simulink library "AVE_Library"  (R2025b)
settings: Solver=VariableStepAuto  StartTime=0.0  StopTime=10.0  RelTol=1e-3
undefined symbols (not defined in the file or in its folder): DiscIntNeverNeededParam
libraries: simulink x44, etargetslib x18, $bdroot x13, GenericTarget x2
(part 3 of 5)

== system AVE_Library/Essential/Signal Logics/Index Of Latest Trigger ==
  vecTrigger : Inport
  Detect Rise Positive : simulink/Logic and Bit Operations/Detect Rise Positive  vinit=0  OutDataTypeStr=boolean
  MATLAB Function : MATLAB Function  TreatAsAtomicUnit=on
  idx : Outport
  wires:
  MATLAB Function/1(value) -> idx/1
  Detect Rise Positive/1 -> MATLAB Function/1(buttons)
  vecTrigger/1 -> Detect Rise Positive/1

== system AVE_Library/Essential/Signal Logics/Index To Enable Vector ==
  idx : Inport  OutDataTypeStr=uint8
  AND : Logic  AllPortsSameDT=off  OutDataTypeStr=boolean
  Cast To Boolean : DataTypeConversion  OutDataTypeStr=boolean  SaturateOnIntegerOverflow=off  RndMeth=Floor
  Compare To Constant : simulink/Logic and Bit Operations/Compare To Constant  relop=<  const=uint8(outputSize)  OutDataTypeStr=boolean
  Compare To Zero : simulink/Logic and Bit Operations/Compare To Zero  relop=>=  OutDataTypeStr=boolean
  Constant43 : Constant  Value=zeros(outputSize,1)  OutDataTypeStr=uint8
  Enabled Subsystem : Subsystem  TreatAsAtomicUnit=on
  Switch : Switch  Criteria=u2 ~= 0  SaturateOnIntegerOverflow=off  InputSameDT=off
  vecEnabled : Outport  OutDataTypeStr=boolean
  wires:
  Cast To Boolean/1 -> vecEnabled/1
  idx/1 -> Compare To Zero/1, Compare To Constant/1, Enabled Subsystem/1(index)
  AND/1 -> Switch/2, Enabled Subsystem/Enable
  Enabled Subsystem/1(vecValue) -> Switch/1
  Compare To Zero/1 -> AND/1
  Switch/1 -> Cast To Boolean/1
  Constant43/1 -> Switch/3
  Compare To Constant/1 -> AND/2

== system AVE_Library/Essential/Signal Logics/Push Buttons To Toggle Switches ==
  pushButtons : Inport  OutDataTypeStr=boolean
  reset : Inport  Port=2  OutDataTypeStr=boolean  PortDimensions=1
  Detect Increase : simulink/Logic and Bit Operations/Detect Increase  vinit=0.0  OutDataTypeStr=boolean
  MATLAB Function : MATLAB Function  TreatAsAtomicUnit=on
  toggleSwitches : Outport  OutDataTypeStr=boolean
  wires:
  Detect Increase/1 -> MATLAB Function/1(riseEvent)
  pushButtons/1 -> Detect Increase/1
  reset/1 -> MATLAB Function/2(resetEvent)
  MATLAB Function/1(output) -> toggleSwitches/1

== system AVE_Library/Essential/Signal Logics/Resetable Index Of Latest Trigger ==
  vecTrigger : Inport
  reset : Inport  Port=2  OutDataTypeStr=boolean  PortDimensions=1
  resetValue : Inport  Port=3  OutDataTypeStr=uint8  PortDimensions=1
  Detect Rise Positive : simulink/Logic and Bit Operations/Detect Rise Positive  vinit=0  OutDataTypeStr=boolean
  MATLAB Function : MATLAB Function  TreatAsAtomicUnit=on
  idx : Outport  OutDataTypeStr=uint8  PortDimensions=1
  wires:
  Detect Rise Positive/1 -> MATLAB Function/1(buttons)
  MATLAB Function/1(value) -> idx/1
  reset/1 -> MATLAB Function/2(reset)
  vecTrigger/1 -> Detect Rise Positive/1
  resetValue/1 -> MATLAB Function/3(resetValue)

== system AVE_Library/Essential/Signal Logics/Resetable Toggle Value Up ==
  triggerUp : Inport  PortDimensions=1
  reset : Inport  Port=2  OutDataTypeStr=boolean  PortDimensions=1
  Detect Rise Positive : simulink/Logic and Bit Operations/Detect Rise Positive  vinit=0  OutDataTypeStr=boolean
  MATLAB Function : MATLAB Function  TreatAsAtomicUnit=on
  value : Outport  OutDataTypeStr=uint8  PortDimensions=1
  wires:
  Detect Rise Positive/1 -> MATLAB Function/1(triggerRise)
  reset/1 -> MATLAB Function/2(reset)
  triggerUp/1 -> Detect Rise Positive/1
  MATLAB Function/1(value) -> value/1

== system AVE_Library/Essential/Signal Logics/Time To Latest Event ==
  event : Inport  OutDataTypeStr=boolean  PortDimensions=1
  steadyClock : Inport  Port=2  OutDataTypeStr=double  Unit=s  PortDimensions=1
  CalculateTimeToLatestEvent : MATLAB Function  TreatAsAtomicUnit=on
  timeToLatestEvent : Outport  OutDataTypeStr=double  Unit=s  PortDimensions=1
  wires:
  event/1 -> CalculateTimeToLatestEvent/1(event)
  steadyClock/1 -> CalculateTimeToLatestEvent/2(t)
  CalculateTimeToLatestEvent/1(timeToLatestEvent) -> timeToLatestEvent/1

== system AVE_Library/Essential/Signal Logics/Toggle Value Up ==
  triggerUp : Inport  PortDimensions=1
  Detect Rise Positive : simulink/Logic and Bit Operations/Detect Rise Positive  vinit=0  OutDataTypeStr=boolean
  Toggle : Subsystem  TreatAsAtomicUnit=on
  value : Outport
  wires:
  Detect Rise Positive/1 -> Toggle/Enable
  triggerUp/1 -> Detect Rise Positive/1
  Toggle/1(value) -> value/1

== system AVE_Library/Essential/Signal Logics/Toggle Value Up Down ==
  triggerUp : Inport  PortDimensions=1
  triggerDown : Inport  Port=2  PortDimensions=1
  Detect Rise Positive1 : simulink/Logic and Bit Operations/Detect Rise Positive  vinit=0  OutDataTypeStr=boolean
  Detect Rise Positive2 : simulink/Logic and Bit Operations/Detect Rise Positive  vinit=0  OutDataTypeStr=boolean
  MATLAB Function : MATLAB Function  TreatAsAtomicUnit=on
  value : Outport  OutDataTypeStr=uint8  PortDimensions=1
  wires:
  triggerUp/1 -> Detect Rise Positive1/1
  Detect Rise Positive2/1 -> MATLAB Function/2(down)
  MATLAB Function/1(y) -> value/1
  triggerDown/1 -> Detect Rise Positive2/1
  Detect Rise Positive1/1 -> MATLAB Function/1(up)

== system AVE_Library/Essential/Signal Logics/Trigger Generator ==
  note: required for safe comparison of doubles
  triggerPeriod : Inport  OutDataTypeStr=double  Unit=s  PortDimensions=1
  reset : Inport  Port=2  OutDataTypeStr=boolean  PortDimensions=1
  Add : Sum  Inputs=-+
  Bias : Bias  Bias=-1.0e-12  SaturateOnIntegerOverflow=off
  Digital Clock : DigitalClock  SampleTime=SampleTime
  Enabled Subsystem : Subsystem  TreatAsAtomicUnit=on
  OR : Logic  Operator=OR  AllPortsSameDT=off  OutDataTypeStr=boolean
  Relational Operator : RelationalOperator  OutDataTypeStr=boolean  RndMeth=Simplest  InputSameDT=off
  Unit Delay : UnitDelay  SampleTime=SampleTime  HasFrameUpgradeWarning=on
  trigger : Outport  OutDataTypeStr=boolean  PortDimensions=1
  wires:
  Unit Delay/1 -> Add/1
  OR/1 -> Enabled Subsystem/Enable, trigger/1
  Enabled Subsystem/1(offsetTime) -> Unit Delay/1  "t0"
  Digital Clock/1 -> Add/2, Enabled Subsystem/1(time)
  Add/1 -> Relational Operator/1
  triggerPeriod/1 -> Bias/1
  Relational Operator/1 -> OR/2
  reset/1 -> OR/1
  Bias/1 -> Relational Operator/2

== system AVE_Library/Essential/Transformation/Euler ZYX To Quaternion ==
  roll : Inport  OutDataTypeStr=double  Unit=rad  PortDimensions=1
  pitch : Inport  Port=2  OutDataTypeStr=double  Unit=rad  PortDimensions=1
  yaw : Inport  Port=3  OutDataTypeStr=double  Unit=rad  PortDimensions=1
  MATLAB Function1 : MATLAB Function  TreatAsAtomicUnit=on
  q_b2n : Outport  OutDataTypeStr=double  PortDimensions=4
  wires:
  yaw/1 -> MATLAB Function1/3(yaw)
  MATLAB Function1/1(q) -> q_b2n/1
  roll/1 -> MATLAB Function1/1(roll)
  pitch/1 -> MATLAB Function1/2(pitch)

== system AVE_Library/Essential/Transformation/Euler ZYX To Rotation Matrix ==
  roll : Inport  OutDataTypeStr=double  Unit=rad  PortDimensions=1
  pitch : Inport  Port=2  OutDataTypeStr=double  Unit=rad  PortDimensions=1
  yaw : Inport  Port=3  OutDataTypeStr=double  Unit=rad  PortDimensions=1
  MATLAB Function : MATLAB Function  TreatAsAtomicUnit=on
  Rb2n : Outport  OutDataTypeStr=double  PortDimensions=[3 3]
  wires:
  yaw/1 -> MATLAB Function/3(yaw)
  MATLAB Function/1(R) -> Rb2n/1
  pitch/1 -> MATLAB Function/2(pitch)
  roll/1 -> MATLAB Function/1(roll)

== system AVE_Library/Essential/Transformation/LLA To NED ==
  lat : Inport  OutDataTypeStr=double  Unit=rad
  lon : Inport  Port=2  OutDataTypeStr=double  Unit=rad
  alt : Inport  Port=3  OutDataTypeStr=double  Unit=m
  originLat : Inport  Port=4  OutDataTypeStr=double  Unit=rad  PortDimensions=1
  originLon : Inport  Port=5  OutDataTypeStr=double  Unit=rad  PortDimensions=1
  originAlt : Inport  Port=6  OutDataTypeStr=double  Unit=m  PortDimensions=1
  MATLAB Function : MATLAB Function  TreatAsAtomicUnit=on
  N : Outport  OutDataTypeStr=double  Unit=m  VectorParamsAs1DForOutWhenUnconnected=off
  E : Outport  Port=2  OutDataTypeStr=double  Unit=m  VectorParamsAs1DForOutWhenUnconnected=off
  D : Outport  Port=3  OutDataTypeStr=double  Unit=m  VectorParamsAs1DForOutWhenUnconnected=off
  wires:
  lon/1 -> MATLAB Function/2(lon)
  originLat/1 -> MATLAB Function/4(originLat)
  MATLAB Function/2(E) -> E/1
  originLon/1 -> MATLAB Function/5(originLon)
  lat/1 -> MATLAB Function/1(lat)
  MATLAB Function/1(N) -> N/1
  alt/1 -> MATLAB Function/3(alt)
  originAlt/1 -> MATLAB Function/6(originAlt)
  MATLAB Function/3(D) -> D/1

== system AVE_Library/Essential/Transformation/LLA To NED Vector ==
  positionLLA : Inport  OutDataTypeStr=double
  originLLA : Inport  Port=2  OutDataTypeStr=double
  MATLAB Function : MATLAB Function  TreatAsAtomicUnit=on
  positionNED : Outport  OutDataTypeStr=double  Unit=m
  wires:
  positionLLA/1 -> MATLAB Function/1(positionLLA)
  MATLAB Function/1(NED) -> positionNED/1
  originLLA/1 -> MATLAB Function/2(originLLA)

== system AVE_Library/Essential/Transformation/NED To LLA ==
  N : Inport  OutDataTypeStr=double  Unit=m
  E : Inport  Port=2  OutDataTypeStr=double  Unit=m
  D : Inport  Port=3  OutDataTypeStr=double  Unit=m
  originLat : Inport  Port=4  OutDataTypeStr=double  Unit=rad  PortDimensions=1
  originLon : Inport  Port=5  OutDataTypeStr=double  Unit=rad  PortDimensions=1
  originAlt : Inport  Port=6  OutDataTypeStr=double  Unit=m  PortDimensions=1
  MATLAB Function : MATLAB Function  TreatAsAtomicUnit=on
  lat : Outport  OutDataTypeStr=double  Unit=rad
  lon : Outport  Port=2  OutDataTypeStr=double  Unit=rad
  alt : Outport  Port=3  OutDataTypeStr=double  Unit=m
  wires:
  MATLAB Function/3(alt) -> alt/1
  MATLAB Function/2(lon) -> lon/1
  MATLAB Function/1(lat) -> lat/1
  N/1 -> MATLAB Function/1(N)
  E/1 -> MATLAB Function/2(E)
  D/1 -> MATLAB Function/3(D)
  originLat/1 -> MATLAB Function/4(originLat)
  originLon/1 -> MATLAB Function/5(originLon)
  originAlt/1 -> MATLAB Function/6(originAlt)

== system AVE_Library/Essential/Transformation/NED To LLA Vector ==
  positionNED : Inport  OutDataTypeStr=double  Unit=m
  originLLA : Inport  Port=2  OutDataTypeStr=double
  MATLAB Function : MATLAB Function  TreatAsAtomicUnit=on
  positionLLA : Outport
  wires:
  positionNED/1 -> MATLAB Function/1(positionNED)
  originLLA/1 -> MATLAB Function/2(originLLA)
  MATLAB Function/1(positionLLA) -> positionLLA/1

== system AVE_Library/Essential/Transformation/Quaternion To Euler ZYX ==
  q_b2n : Inport  OutDataTypeStr=double  PortDimensions=4
  MATLAB Function : MATLAB Function  TreatAsAtomicUnit=on
  roll : Outport  OutDataTypeStr=double  Unit=rad  PortDimensions=1
  pitch : Outport  Port=2  OutDataTypeStr=double  Unit=rad  PortDimensions=1
  yaw : Outport  Port=3  OutDataTypeStr=double  Unit=rad  PortDimensions=1
  wires:
  MATLAB Function/1(roll) -> roll/1
  q_b2n/1 -> MATLAB Function/1(q)
  MATLAB Function/3(yaw) -> yaw/1
  MATLAB Function/2(pitch) -> pitch/1

== system AVE_Library/Essential/Transformation/Quaternion To Rotation Matrix ==
  q_b2n : Inport  OutDataTypeStr=double  PortDimensions=4
  MATLAB Function : MATLAB Function  TreatAsAtomicUnit=on
  Cb2n : Outport  OutDataTypeStr=double
  wires:
  q_b2n/1 -> MATLAB Function/1(qb2n)
  MATLAB Function/1(matCb2n) -> Cb2n/1

== system AVE_Library/Essential/Transformation/Transform Sensor Euler ZYX ==
  rollSensor : Inport  OutDataTypeStr=double  Unit=rad  PortDimensions=1
  pitchSensor : Inport  Port=2  OutDataTypeStr=double  Unit=rad  PortDimensions=1
  yawSensor : Inport  Port=3  OutDataTypeStr=double  Unit=rad  PortDimensions=1
  R_b2s : Inport  Port=4  OutDataTypeStr=double  PortDimensions=[3 3]
  MATLAB Function : MATLAB Function  TreatAsAtomicUnit=on
  rollBody : Outport  OutDataTypeStr=double  Unit=rad  PortDimensions=1
  pitchBody : Outport  Port=2  OutDataTypeStr=double  Unit=rad  PortDimensions=1
  yawBody : Outport  Port=3  OutDataTypeStr=double  Unit=rad  PortDimensions=1
  wires:
  rollSensor/1 -> MATLAB Function/1(rollSensor)
  MATLAB Function/2(pitchBody) -> pitchBody/1
  R_b2s/1 -> MATLAB Function/4(R_b2s)
  MATLAB Function/1(rollBody) -> rollBody/1
  pitchSensor/1 -> MATLAB Function/2(pitchSensor)
  yawSensor/1 -> MATLAB Function/3(yawSensor)
  MATLAB Function/3(yawBody) -> yawBody/1

== system AVE_Library/Essential/Transformation/Transform Sensor Position LLA ==
  latSensor : Inport  OutDataTypeStr=double  Unit=rad  PortDimensions=1
  lonSensor : Inport  Port=2  OutDataTypeStr=double  Unit=rad  PortDimensions=1
  altSensor : Inport  Port=3  OutDataTypeStr=double  Unit=m  PortDimensions=1
  R_b2n : Inport  Port=4  OutDataTypeStr=double  PortDimensions=[3 3]
  r_b2s : Inport  Port=5  OutDataTypeStr=double  PortDimensions=3
  MATLAB Function : MATLAB Function  TreatAsAtomicUnit=on
  latBody : Outport  OutDataTypeStr=double  Unit=rad  PortDimensions=1
  lonBody : Outport  Port=2  OutDataTypeStr=double  Unit=rad  PortDimensions=1
  altBody : Outport  Port=3  OutDataTypeStr=double  Unit=m  PortDimensions=1
  wires:
  altSensor/1 -> MATLAB Function/3(altSensor)
  MATLAB Function/3(altBody) -> altBody/1
  MATLAB Function/2(lonBody) -> lonBody/1
  MATLAB Function/1(latBody) -> latBody/1
  latSensor/1 -> MATLAB Function/1(latSensor)
  lonSensor/1 -> MATLAB Function/2(lonSensor)
  R_b2n/1 -> MATLAB Function/4(R_b2n)
  r_b2s/1 -> MATLAB Function/5(r_b2s)

== system AVE_Library/Essential/Transformation/Transform Sensor Quaternion WXYZ ==
  quaternionSensor : Inport  OutDataTypeStr=double  PortDimensions=4
  R_b2s : Inport  Port=2  OutDataTypeStr=double  PortDimensions=[3 3]
  MATLAB Function : MATLAB Function  TreatAsAtomicUnit=on
  quaternionBody : Outport  OutDataTypeStr=double  PortDimensions=4
  wires:
  MATLAB Function/1(quaternionBody) -> quaternionBody/1
  quaternionSensor/1 -> MATLAB Function/1(quaternionSensor)
  R_b2s/1 -> MATLAB Function/2(R_b2s)

== system AVE_Library/Essential/Transformation/Transform Sensor Velocity PQR ==
  pSensor : Inport  OutDataTypeStr=double  Unit=rad/s  PortDimensions=1
  qSensor : Inport  Port=2  OutDataTypeStr=double  Unit=rad/s  PortDimensions=1
  rSensor : Inport  Port=3  OutDataTypeStr=double  Unit=rad/s  PortDimensions=1
  R_b2s : Inport  Port=4  OutDataTypeStr=double  PortDimensions=[3 3]
  MATLAB Function : MATLAB Function  TreatAsAtomicUnit=on
  pBody : Outport  OutDataTypeStr=double  Unit=rad/s  PortDimensions=1
  qBody : Outport  Port=2  OutDataTypeStr=double  Unit=rad/s  PortDimensions=1
  rBody : Outport  Port=3  OutDataTypeStr=double  Unit=rad/s  PortDimensions=1
  wires:
  MATLAB Function/3(rBody) -> rBody/1
  rSensor/1 -> MATLAB Function/3(rSensor)
  qSensor/1 -> MATLAB Function/2(qSensor)
  MATLAB Function/1(pBody) -> pBody/1
  R_b2s/1 -> MATLAB Function/4(R_b2s)
  MATLAB Function/2(qBody) -> qBody/1
  pSensor/1 -> MATLAB Function/1(pSensor)

== system AVE_Library/Essential/Transformation/Transform Sensor Velocity UVW ==
  uSensor : Inport  OutDataTypeStr=double  Unit=m/s  PortDimensions=1
  vSensor : Inport  Port=2  OutDataTypeStr=double  Unit=m/s  PortDimensions=1
  wSensor : Inport  Port=3  OutDataTypeStr=double  Unit=m/s  PortDimensions=1
  R_b2s : Inport  Port=4  OutDataTypeStr=double  PortDimensions=[3 3]
  r_b2s : Inport  Port=5  OutDataTypeStr=double  Unit=m  PortDimensions=3
  pqr : Inport  Port=6  OutDataTypeStr=double  Unit=rad/s  PortDimensions=3
  MATLAB Function : MATLAB Function  TreatAsAtomicUnit=on
  uBody : Outport  OutDataTypeStr=double  Unit=m/s  PortDimensions=1
  vBody : Outport  Port=2  OutDataTypeStr=double  Unit=m/s  PortDimensions=1
  wBody : Outport  Port=3  OutDataTypeStr=double  Unit=m/s  PortDimensions=1
  wires:
  uSensor/1 -> MATLAB Function/1(uSensor)
  MATLAB Function/2(vBody) -> vBody/1
  R_b2s/1 -> MATLAB Function/4(R_b2s)
  MATLAB Function/1(uBody) -> uBody/1
  pqr/1 -> MATLAB Function/6(pqr)
  vSensor/1 -> MATLAB Function/2(vSensor)
  r_b2s/1 -> MATLAB Function/5(r_b2s)
  wSensor/1 -> MATLAB Function/3(wSensor)
  MATLAB Function/3(wBody) -> wBody/1

== system AVE_Library/Essential/Transformation/Yaw To Rotation Matrix ==
  yaw : Inport  OutDataTypeStr=double  Unit=rad  PortDimensions=1
  MATLAB Function : MATLAB Function  TreatAsAtomicUnit=on
  Rb2n : Outport  OutDataTypeStr=double  PortDimensions=[2 2]
  wires:
  MATLAB Function/1(R) -> Rb2n/1
  yaw/1 -> MATLAB Function/1(yaw)

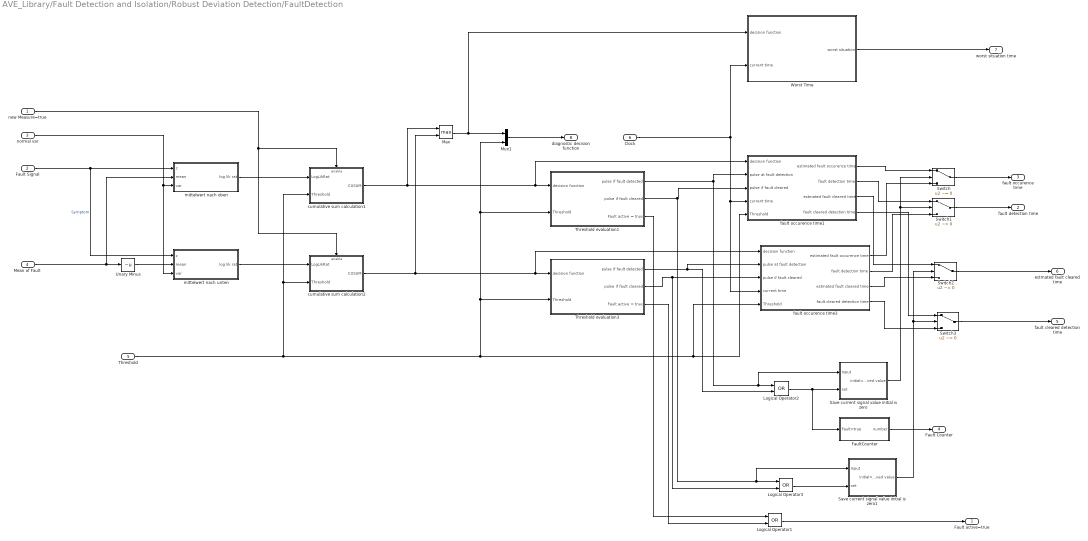
== system AVE_Library/Fault Detection and Isolation/Robust Deviation Detection/FaultDetection ==
  new Measure=true : Inport
  Fault Signal : Inport  Port=2
  normal var : Inport  Port=3
  Mean of Fault : Inport  Port=4
  Threshold : Inport  Port=5
  Clock : Inport  Port=6
  FaultCounter : Subsystem
  Logical Operator1 : Logic  Operator=OR  AllPortsSameDT=off  OutDataTypeStr=boolean
  Logical Operator2 : Logic  Operator=OR  AllPortsSameDT=off  OutDataTypeStr=boolean
  Logical Operator3 : Logic  Operator=OR  AllPortsSameDT=off  OutDataTypeStr=boolean
  Max : MinMax  Function=max  Inputs=2
  Mux1 : Mux  Inputs=2
  Save current signal value initial is zero : Subsystem  mask(save current signal value){}
      mask help:
      | If set is not zero, the input is feed throug to the output.
      | If set is zero, the output remains the last intput value when set was not zero.
      | Initial value is zero.
  Save current signal value initial is zero1 : Subsystem  mask(save current signal value){}
      mask help:
      | If set is not zero, the input is feed throug to the output.
      | If set is zero, the output remains the last intput value when set was not zero.
      | Initial value is zero.
  Switch{,1..3} (4 alike) : Switch  Criteria=u2 ~= 0  SaturateOnIntegerOverflow=off  InputSameDT=off
  Threshold evaluation1 : Subsystem
  Threshold evaluation3 : Subsystem
  Unary Minus : UnaryMinus
  Worst Time : Subsystem
  cumulative sum calculation1 : Subsystem
  cumulative sum calculation2 : Subsystem
  fault occurence time1 : Subsystem
  fault occurence time3 : Subsystem
  mittelwert nach oben : Subsystem
  mittelwert nach unten : Subsystem
  Fault active=true : Outport  VectorParamsAs1DForOutWhenUnconnected=off
  fault detection time : Outport  Port=2  VectorParamsAs1DForOutWhenUnconnected=off
  fault occurence time : Outport  Port=3  VectorParamsAs1DForOutWhenUnconnected=off
  Fault Counter : Outport  Port=4  VectorParamsAs1DForOutWhenUnconnected=off
  fault cleared detection time : Outport  Port=5  VectorParamsAs1DForOutWhenUnconnected=off
  estmated fault cleared time : Outport  Port=6  VectorParamsAs1DForOutWhenUnconnected=off
  worst situation time : Outport  Port=7  VectorParamsAs1DForOutWhenUnconnected=off
  diagnostic decision function : Outport  Port=8  VectorParamsAs1DForOutWhenUnconnected=off
  wires:
  mittelwert nach unten/1(log lik rat) -> cumulative sum calculation2/1(LogLikRat)
  mittelwert nach oben/1(log lik rat) -> cumulative sum calculation1/1(LogLikRat)
  Worst Time/1(worst situation) -> worst situation time/1
  Switch3/1 -> fault cleared detection time/1
  Switch2/1 -> estmated fault cleared time/1
  fault occurence time3/3(estmated fault cleared time) -> Switch2/3
  fault occurence time3/4(fault cleared detection time) -> Switch3/3
  fault occurence time1/4(fault cleared detection time) -> Switch3/1
  fault occurence time1/3(estmated fault cleared time) -> Switch2/1
  Save current signal value initial is zero1/1(initial=0  saved value) -> Switch3/2, Switch2/2
  Threshold evaluation1/2(pulse if fault cleared) -> fault occurence time1/3(pulse if fault cleared), Logical Operator3/1, Save current signal value initial is zero1/1(Input)
  Logical Operator3/1 -> Save current signal value initial is zero1/2(set)
  Threshold evaluation3/2(pulse if fault cleared) -> Logical Operator3/2, fault occurence time3/3(pulse if fault cleared)
  FaultCounter/1(number) -> Fault Counter/1
  Mux1/1 -> diagnostic decision function/1
  Threshold/1 -> cumulative sum calculation2/2(Threshold), cumulative sum calculation1/2(Threshold), Mux1/2, Threshold evaluation1/2(Threshold), Threshold evaluation3/2(Threshold), fault occurence time1/5(Threshold), fault occurence time3/5(Threshold)
  Max/1 -> Mux1/1, Worst Time/1(decision function)
  Logical Operator1/1 -> Fault active=true/1
  fault occurence time3/2(fault detection time) -> Switch1/3
  fault occurence time1/2(fault detection time) -> Switch1/1
  fault occurence time3/1(estimated fault occurence time) -> Switch/3
  fault occurence time1/1(estimated fault occurence time) -> Switch/1
  Threshold evaluation3/3(Fault active = true) -> Logical Operator1/2
  Threshold evaluation1/3(Fault active = true) -> Logical Operator1/1
  Threshold evaluation3/1(pulse if fault detected) -> Logical Operator2/2, fault occurence time3/2(pulse at fault detection)
  new Measure=true/1 -> cumulative sum calculation1/Enable, cumulative sum calculation2/Enable
  cumulative sum calculation2/1(CUSUM) -> Max/2, fault occurence time3/1(decision function), Threshold evaluation3/1(decision function)
  Save current signal value initial is zero/1(initial=0  saved value) -> Switch1/2, Switch/2
  Logical Operator2/1 -> Save current signal value initial is zero/2(set), FaultCounter/1(Fault=true)
  Threshold evaluation1/1(pulse if fault detected) -> fault occurence time1/2(pulse at fault detection), Save current signal value initial is zero/1(Input), Logical Operator2/1
  Switch1/1 -> fault detection time/1
  Switch/1 -> fault occurence time/1
  cumulative sum calculation1/1(CUSUM) -> Max/1, fault occurence time1/1(decision function), Threshold evaluation1/1(decision function)
  Unary Minus/1 -> mittelwert nach unten/2(mean)
  Clock/1 -> fault occurence time1/4(current time), fault occurence time3/4(current time), Worst Time/2(current time)
  Mean of Fault/1 -> Unary Minus/1, mittelwert nach oben/2(mean)
  Fault Signal/1 -> mittelwert nach unten/1(z), mittelwert nach oben/1(z)  "Symptom"
  normal var/1 -> mittelwert nach oben/3(var), mittelwert nach unten/3(var)

== system AVE_Library/Fault Detection and Isolation/Robust Deviation Detection/mittelwert nach oben ==
  mean : Inport
  z : Inport  Port=2
  var : Inport  Port=3
  Gain2 : Gain  Gain=0.5
  Product1 : Product  Inputs=**/  RndMeth=Zero
  Sum : Sum  Inputs=+-|
  null Vermeiden : Subsystem  mask{kleinsterWert=1e-8}
      mask prompts: kleinsterWert "Null-Mindestabstand"
      mask help:
      | Der Ausgang hält einen vorgegebenen Abstand zu Null.
      | Wenn der Eingang einen Nulldurchlauf hat, springt der Ausgang von +Mindestabstand nach -Mindestabstand, bzw. von -Mindestabstand nach +Mindestabstand. Bei Eingang ==0: Ausgang=+Mindestabstand
  log lik rat : Outport  VectorParamsAs1DForOutWhenUnconnected=off
  wires:
  null Vermeiden/1(non zero) -> Product1/3
  Gain2/1 -> Sum/2
  Sum/1 -> Product1/1
  z/1 -> Sum/1
  Product1/1 -> log lik rat/1
  var/1 -> null Vermeiden/1(value)
  mean/1 -> Gain2/1, Product1/2

== system AVE_Library/Fault Detection and Isolation/Robust Deviation Detection/statistics ==
  measurement value : Inport
  measurement state 1/0 : Inport  Port=2
  n max : Inport  Port=3
  Constant1 : Constant  Value=0
  Messwertzähler : Subsystem
  Subsystem : Subsystem
  var : Outport
  wires:
  measurement state 1/0/1 -> Messwertzähler/1(measurement state), Subsystem/Enable
  Constant1/1 -> Subsystem/1(mean)
  n max/1 -> Messwertzähler/2(n max)
  Messwertzähler/1(number) -> Subsystem/2(n measurements)
  measurement value/1 -> Subsystem/3(measurement)
  Subsystem/1(var) -> var/1

== system AVE_Library/Navigation/Sensor Preprocessing/Butterworth Filter ==
  u : Inport
  T : Inport  Port=2
  Butterworth Low Pass and Derivation : Subsystem  mask(Butterworth Lowpass Filter){n_Ordnung_Butter_Simulink=numPoles, n_Ableitung=numZeros}
      mask prompts: n_Ordnung_Butter_Simulink "Ordnung Tiefpass"; n_Ableitung "Anzahl Ableitungen"
      mask help:
      | Butterworth Lowpass Filter mit variabler Frequenz.
      | Ordnung ist nicht online tunable, dies würde zu variabler Dimension der Matrizen führen.
      mask init:
      | if n_Ableitung==0
      |     nozerosFlag=1;
      |     Nullstellen=0;
      | else
      |     nozerosFlag=0;
      |     Nullstellen=zeros(1,n_Ableitung);
      | end
      | 
      | 
      | if n_Ableitung>n_Ordnung_Butter_Simulink
      |     error('Ordnung muss mindestens so hoch wie Anzahl Ableitungen sein. ')
      | end
      mask Display:
      | %text(.5,.5,'{\itEquation:}  \Sigma \alpha^2 + \beta^2 \rightarrow \infty, \Pi, \phi_3 = {\bfcool}', 'hor','left','texmode','on')
      | %text(0.5, 0.5, ['Butterworth\nLowpass\n n_Ordnung=' num2str(n_Ordnung_Butter_Simulink) '\nn_Ableitungen=' num2str(n_Ableitung) ], 'horizontalAlignment', 'center');
      | text(0.5, 0.5, 'Butterworth\nFilter Design', 'horizontalAlignment', 'center');
  Detect Change : simulink/Logic and Bit Operations/Detect Change  vinit=0  OutDataTypeStr=boolean
  Zustandsraummodell x0=x_t_inf(u=u_t_0) : Subsystem
  y : Outport  VectorParamsAs1DForOutWhenUnconnected=off
  wires:
  Detect Change/1 -> Zustandsraummodell x0=x_t_inf(u=u_t_0)/6(reset)
  T/1 -> Detect Change/1, Butterworth Low Pass and Derivation/1(T)
  Butterworth Low Pass and Derivation/2(B) -> Zustandsraummodell x0=x_t_inf(u=u_t_0)/2(B)
  Zustandsraummodell x0=x_t_inf(u=u_t_0)/1(y) -> y/1
  Butterworth Low Pass and Derivation/4(D) -> Zustandsraummodell x0=x_t_inf(u=u_t_0)/4(D)
  Butterworth Low Pass and Derivation/1(A) -> Zustandsraummodell x0=x_t_inf(u=u_t_0)/1(A)
  Butterworth Low Pass and Derivation/3(C) -> Zustandsraummodell x0=x_t_inf(u=u_t_0)/3(C)
  u/1 -> Zustandsraummodell x0=x_t_inf(u=u_t_0)/5(u)

== system AVE_Library/Navigation/Sensor Preprocessing/Detect Outliers 1D ==
  triggerNewData : Inport  OutDataTypeStr=boolean  PortDimensions=1
  data : Inport  Port=2  OutDataTypeStr=double  PortDimensions=1
  threshold : Inport  Port=3  OutDataTypeStr=double  PortDimensions=1
  maxNumOutliers : Inport  Port=4  OutDataTypeStr=uint32  PortDimensions=1
  Abs2 : Abs  SaturateOnIntegerOverflow=off
  Constant : Constant  OutDataTypeStr=uint32
  MATLAB Function : MATLAB Function  TreatAsAtomicUnit=on
  Max : MinMax  Function=max  Inputs=2
  numberOfOutliers : Outport  OutDataTypeStr=uint32  PortDimensions=1
  wires:
  MATLAB Function/1(numberOfOutliers) -> numberOfOutliers/1
  data/1 -> MATLAB Function/2(data)
  triggerNewData/1 -> MATLAB Function/1(triggerNewData)
  threshold/1 -> Abs2/1
  Abs2/1 -> MATLAB Function/3(threshold)
  Constant/1 -> Max/2
  maxNumOutliers/1 -> Max/1
  Max/1 -> MATLAB Function/4(maxNumOutliers)

== system AVE_Library/Navigation/Sensor Preprocessing/Detect Outliers Angle 1D ==
  triggerNewData : Inport  OutDataTypeStr=boolean  PortDimensions=1
  data : Inport  Port=2  OutDataTypeStr=double  PortDimensions=1
  threshold : Inport  Port=3  OutDataTypeStr=double  PortDimensions=1
  maxNumOutliers : Inport  Port=4  OutDataTypeStr=uint32  PortDimensions=1
  Abs2 : Abs  SaturateOnIntegerOverflow=off
  Constant : Constant  OutDataTypeStr=uint32
  MATLAB Function : MATLAB Function  TreatAsAtomicUnit=on
  Max : MinMax  Function=max  Inputs=2
  numberOfOutliers : Outport  OutDataTypeStr=uint32  PortDimensions=1
  wires:
  Max/1 -> MATLAB Function/4(maxNumOutliers)
  maxNumOutliers/1 -> Max/1
  Constant/1 -> Max/2
  Abs2/1 -> MATLAB Function/3(threshold)
  threshold/1 -> Abs2/1
  triggerNewData/1 -> MATLAB Function/1(triggerNewData)
  data/1 -> MATLAB Function/2(data)
  MATLAB Function/1(numberOfOutliers) -> numberOfOutliers/1

== system AVE_Library/Navigation/Sensor Preprocessing/Detect Outliers GNSS ==
  triggerNewData : Inport  OutDataTypeStr=boolean  PortDimensions=1
  positionLLA : Inport  Port=2  OutDataTypeStr=double  PortDimensions=3
  thresholdHorizontal : Inport  Port=3  OutDataTypeStr=double  Unit=m  PortDimensions=1
  thresholdVertical : Inport  Port=4  OutDataTypeStr=double  Unit=m  PortDimensions=1
  maxNumOutliers : Inport  Port=5  OutDataTypeStr=uint32  PortDimensions=1
  Abs1 : Abs  SaturateOnIntegerOverflow=off
  Abs2 : Abs  SaturateOnIntegerOverflow=off
  Constant : Constant  OutDataTypeStr=uint32
  MATLAB Function : MATLAB Function  TreatAsAtomicUnit=on
  Max : MinMax  Function=max  Inputs=2
  numberOfOutliers : Outport  OutDataTypeStr=uint32  PortDimensions=1
  wires:
  Max/1 -> MATLAB Function/5(maxNumOutliers)
  maxNumOutliers/1 -> Max/1
  Constant/1 -> Max/2
  Abs2/1 -> MATLAB Function/3(thresholdHorizontal)
  thresholdHorizontal/1 -> Abs2/1
  triggerNewData/1 -> MATLAB Function/1(triggerNewData)
  positionLLA/1 -> MATLAB Function/2(positionLLA)
  MATLAB Function/1(numberOfOutliers) -> numberOfOutliers/1
  Abs1/1 -> MATLAB Function/4(thresholdVertical)
  thresholdVertical/1 -> Abs1/1

== system AVE_Library/Navigation/Sensor Preprocessing/Smoothed Quaternion Time Derivative ==
  time : Inport  OutDataTypeStr=double  Unit=s  PortDimensions=1
  trigger : Inport  Port=2  OutDataTypeStr=boolean  PortDimensions=1
  q_b2n : Inport  Port=3  OutDataTypeStr=double  PortDimensions=4
  timeconstant : Inport  Port=4  OutDataTypeStr=double  Unit=s  PortDimensions=1
  Demux : Demux
  Mux : Mux  Inputs=3
  SmoothedOrientationDeviation : MATLAB Function  TreatAsAtomicUnit=on
  pqr : Outport  OutDataTypeStr=double  Unit=rad/s  PortDimensions=3
  wires:
  time/1 -> SmoothedOrientationDeviation/1(time)
  timeconstant/1 -> SmoothedOrientationDeviation/7(T)
  trigger/1 -> SmoothedOrientationDeviation/2(trigger)
  SmoothedOrientationDeviation/2(q) -> Mux/2
  SmoothedOrientationDeviation/1(p) -> Mux/1
  SmoothedOrientationDeviation/3(r) -> Mux/3
  Mux/1 -> pqr/1
  q_b2n/1 -> Demux/1
  Demux/1 -> SmoothedOrientationDeviation/3(qw)
  Demux/2 -> SmoothedOrientationDeviation/4(qx)
  Demux/3 -> SmoothedOrientationDeviation/5(qy)
  Demux/4 -> SmoothedOrientationDeviation/6(qz)

== system AVE_Library/Navigation/Sensor Preprocessing/Triggered Low Pass ==
  time : Inport  OutDataTypeStr=double  Unit=s  PortDimensions=1
  trigger : Inport  Port=2  OutDataTypeStr=boolean  PortDimensions=1
  input : Inport  Port=3  OutDataTypeStr=double
  timeconstant : Inport  Port=4  OutDataTypeStr=double  Unit=s  PortDimensions=1
  TriggeredLowPass : MATLAB Function  TreatAsAtomicUnit=on
  output : Outport  OutDataTypeStr=double
  wires:
  time/1 -> TriggeredLowPass/1(time)
  input/1 -> TriggeredLowPass/3(u)
  timeconstant/1 -> TriggeredLowPass/4(T)
  trigger/1 -> TriggeredLowPass/2(trigger)
  TriggeredLowPass/1(y) -> output/1

== system AVE_Library/Essential/Equations of Motion/Kinematic 6DoF Geographic/Enabled Subsystem ==
  In1 : Inport
  Enable : EnablePort
  Out1 : Outport  VectorParamsAs1DForOutWhenUnconnected=off
  wires:
  In1/1 -> Out1/1

== system AVE_Library/Essential/Network/Swap Double Host To Network/Swap Each Element ==
  in : Inport  Partition=on  PartitionDimension=1  PartitionWidth=1  PartitionOffset=0
  Byte Pack : etargetslib/Byte Pack  datatypes={'double'}  byteAlign=1
  Byte Unpack : etargetslib/Byte Unpack  dimensions={[1]}  datatypes={'double'}  byteAlign=1
  For Each : ForEach  DisableCoverage=on
  Selector : Selector  InputPortWidth=8  IndexOptions=Index vector (dialog)  Indices=[8 7 6 5 4 3 2 1]  OutputSizes=1
  out : Outport  ConcatenationDimension=1
  wires:
  Selector/1 -> Byte Unpack/1
  Byte Pack/1 -> Selector/1
  Byte Unpack/1 -> out/1
  in/1 -> Byte Pack/1

== system AVE_Library/Essential/Network/Swap Float Host To Network/Swap Each Element ==
  in : Inport  Partition=on  PartitionDimension=1  PartitionWidth=1  PartitionOffset=0
  Byte Pack : etargetslib/Byte Pack  datatypes={'single'}  byteAlign=1
  Byte Unpack : etargetslib/Byte Unpack  dimensions={[1]}  datatypes={'single'}  byteAlign=1
  For Each : ForEach  DisableCoverage=on
  Selector : Selector  InputPortWidth=4  IndexOptions=Index vector (dialog)  Indices=[4 3 2 1]  OutputSizes=1
  out : Outport  ConcatenationDimension=1
  wires:
  Selector/1 -> Byte Unpack/1
  Byte Pack/1 -> Selector/1
  Byte Unpack/1 -> out/1
  in/1 -> Byte Pack/1

== system AVE_Library/Essential/Network/Swap Int16 Host To Network/Swap Each Element ==
  in : Inport  Partition=on  PartitionDimension=1  PartitionWidth=1  PartitionOffset=0
  Byte Pack : etargetslib/Byte Pack  datatypes={'int16'}  byteAlign=1
  Byte Unpack : etargetslib/Byte Unpack  dimensions={[1]}  datatypes={'int16'}  byteAlign=1
  For Each : ForEach  DisableCoverage=on
  Selector : Selector  InputPortWidth=2  IndexOptions=Index vector (dialog)  Indices=[2 1]  OutputSizes=1
  out : Outport  ConcatenationDimension=1
  wires:
  Selector/1 -> Byte Unpack/1
  Byte Pack/1 -> Selector/1
  Byte Unpack/1 -> out/1
  in/1 -> Byte Pack/1

== system AVE_Library/Essential/Network/Swap Int32 Host To Network/Swap Each Element ==
  in : Inport  Partition=on  PartitionDimension=1  PartitionWidth=1  PartitionOffset=0
  Byte Pack : etargetslib/Byte Pack  datatypes={'int32'}  byteAlign=1
  Byte Unpack : etargetslib/Byte Unpack  dimensions={[1]}  datatypes={'int32'}  byteAlign=1
  For Each : ForEach  DisableCoverage=on
  Selector : Selector  InputPortWidth=4  IndexOptions=Index vector (dialog)  Indices=[4 3 2 1]  OutputSizes=1
  out : Outport  ConcatenationDimension=1
  wires:
  Selector/1 -> Byte Unpack/1
  Byte Pack/1 -> Selector/1
  Byte Unpack/1 -> out/1
  in/1 -> Byte Pack/1

== system AVE_Library/Essential/Network/Swap Uint16 Host To Network/Swap Each Element ==
  in : Inport  Partition=on  PartitionDimension=1  PartitionWidth=1  PartitionOffset=0
  Byte Pack : etargetslib/Byte Pack  datatypes={'uint16'}  byteAlign=1
  Byte Unpack : etargetslib/Byte Unpack  dimensions={[1]}  datatypes={'uint16'}  byteAlign=1
  For Each : ForEach  DisableCoverage=on
  Selector : Selector  InputPortWidth=2  IndexOptions=Index vector (dialog)  Indices=[2 1]  OutputSizes=1
  out : Outport  ConcatenationDimension=1
  wires:
  Selector/1 -> Byte Unpack/1
  Byte Pack/1 -> Selector/1
  Byte Unpack/1 -> out/1
  in/1 -> Byte Pack/1

== system AVE_Library/Essential/Network/Swap Uint32 Host To Network/Swap Each Element ==
  in : Inport  Partition=on  PartitionDimension=1  PartitionWidth=1  PartitionOffset=0
  Byte Pack : etargetslib/Byte Pack  datatypes={'uint32'}  byteAlign=1
  Byte Unpack : etargetslib/Byte Unpack  dimensions={[1]}  datatypes={'uint32'}  byteAlign=1
  For Each : ForEach  DisableCoverage=on
  Selector : Selector  InputPortWidth=4  IndexOptions=Index vector (dialog)  Indices=[4 3 2 1]  OutputSizes=1
  out : Outport  ConcatenationDimension=1
  wires:
  in/1 -> Byte Pack/1
  Byte Unpack/1 -> out/1
  Byte Pack/1 -> Selector/1
  Selector/1 -> Byte Unpack/1

== system AVE_Library/Essential/Signal Logics/Index To Enable Vector/Enabled Subsystem ==
  index : Inport
  Enable : EnablePort
  Assignment : Assignment  IndexMode=Zero-based  DiagnosticForDimensions=Warning  IndexOptions=Index vector (port)  Indices=1  OutputSizes=1
  Constant43 : Constant  Value=zeros(outputSize,1)  OutDataTypeStr=uint8
  Constant44 : Constant  OutDataTypeStr=uint8
  vecValue : Outport
  wires:
  Assignment/1 -> vecValue/1
  Constant43/1 -> Assignment/1
  index/1 -> Assignment/3
  Constant44/1 -> Assignment/2

== system AVE_Library/Essential/Signal Logics/Toggle Value Up/Toggle ==
  Enable : EnablePort
  Bias : Bias  Bias=uint8(1)  SaturateOnIntegerOverflow=off
  Compare To Constant : simulink/Logic and Bit Operations/Compare To Constant  relop=<=  const=uint8(maxValue)  OutDataTypeStr=boolean
  Constant : Constant  Value=0  OutDataTypeStr=uint8
  Switch : Switch  Criteria=u2 ~= 0  SaturateOnIntegerOverflow=off  InputSameDT=off
  Unit Delay : UnitDelay  InitialCondition=uint8(0)  SampleTime=-1  HasFrameUpgradeWarning=on
  value : Outport  OutDataTypeStr=uint8  PortDimensions=1
  wires:
  Switch/1 -> Unit Delay/1, value/1
  Constant/1 -> Switch/3
  Compare To Constant/1 -> Switch/2
  Bias/1 -> Switch/1, Compare To Constant/1
  Unit Delay/1 -> Bias/1

== system AVE_Library/Essential/Signal Logics/Trigger Generator/Enabled Subsystem ==
  time : Inport
  Enable : EnablePort
  offsetTime : Outport
  wires:
  time/1 -> offsetTime/1

== system AVE_Library/Fault Detection and Isolation/Robust Deviation Detection/FaultDetection/FaultCounter ==
  Fault=true : Inport
  Data Type Conversion : DataTypeConversion  OutDataTypeStr=uint32  SaturateOnIntegerOverflow=off  RndMeth=Floor
  Memory : Memory  InheritSampleTime=on
  Sum : Sum  Inputs=|++
  number : Outport
  wires:
  Memory/1 -> Sum/1
  Sum/1 -> Memory/1, number/1
  Fault=true/1 -> Data Type Conversion/1
  Data Type Conversion/1 -> Sum/2

== system AVE_Library/Fault Detection and Isolation/Robust Deviation Detection/FaultDetection/Save current signal value initial is zero ==
  Input : Inport
  set : Inport  Port=2
  Init : Switch  Criteria=u2 ~= 0  OutDataTypeStr=Inherit: Inherit via back propagation  ZeroCross=off  SaturateOnIntegerOverflow=off  InputSameDT=off
  Memory : Memory  InheritSampleTime=on
  Reset : Switch  Criteria=u2 ~= 0  OutDataTypeStr=Inherit: Inherit via back propagation  ZeroCross=off  SaturateOnIntegerOverflow=off  InputSameDT=off
  initial=0  saved value : Outport  VectorParamsAs1DForOutWhenUnconnected=off
  wires:
  set/1 -> Reset/2, Init/2
  Memory/1 -> Init/3
  Init/1 -> initial=0  saved value/1, Reset/3
  Reset/1 -> Memory/1
  Input/1 -> Reset/1, Init/1

== system AVE_Library/Fault Detection and Isolation/Robust Deviation Detection/FaultDetection/Save current signal value initial is zero1 ==
  Input : Inport
  set : Inport  Port=2
  Init : Switch  Criteria=u2 ~= 0  OutDataTypeStr=Inherit: Inherit via back propagation  ZeroCross=off  SaturateOnIntegerOverflow=off  InputSameDT=off
  Memory : Memory  InheritSampleTime=on
  Reset : Switch  Criteria=u2 ~= 0  OutDataTypeStr=Inherit: Inherit via back propagation  ZeroCross=off  SaturateOnIntegerOverflow=off  InputSameDT=off
  initial=0  saved value : Outport  VectorParamsAs1DForOutWhenUnconnected=off
  wires:
  Input/1 -> Init/1, Reset/1
  Reset/1 -> Memory/1
  Init/1 -> Reset/3, initial=0  saved value/1
  Memory/1 -> Init/3
  set/1 -> Init/2, Reset/2

== system AVE_Library/Fault Detection and Isolation/Robust Deviation Detection/FaultDetection/Threshold evaluation1 ==
  decision function : Inport
  Threshold : Inport  Port=2
  Compare To Zero : simulink/Logic and Bit Operations/Compare To Zero  relop===  OutDataTypeStr=boolean
  Detect Decrease : simulink/Logic and Bit Operations/Detect Decrease  vinit=0.0  OutDataTypeStr=boolean
  Detect Increase : simulink/Logic and Bit Operations/Detect Increase  vinit=0.0  OutDataTypeStr=boolean
  Detect Increase1 : simulink/Logic and Bit Operations/Detect Increase  vinit=0.0  OutDataTypeStr=boolean
  Detect Increase2 : simulink/Logic and Bit Operations/Detect Increase  vinit=0.0  OutDataTypeStr=boolean
  FehlerSpeicher : Subsystem  mask(save current signal value){}
      mask help:
      | If set is not zero, the input is feed throug to the output.
      | If set is zero, the output remains the last intput value when set was not zero.
      | Initial value is zero.
  OR : Logic  Operator=OR  AllPortsSameDT=off  OutDataTypeStr=boolean
  decisionfunction crosses threshold : RelationalOperator  OutDataTypeStr=boolean  InputSameDT=off
  pulse if fault detected : Outport  VectorParamsAs1DForOutWhenUnconnected=off
  pulse if fault cleared : Outport  Port=2  VectorParamsAs1DForOutWhenUnconnected=off
  Fault active = true : Outport  Port=3  VectorParamsAs1DForOutWhenUnconnected=off
  wires:
  Detect Decrease/1 -> pulse if fault cleared/1
  Detect Increase2/1 -> pulse if fault detected/1
  FehlerSpeicher/1(initial=0  saved value) -> Detect Increase2/1, Detect Decrease/1, Fault active = true/1
  Detect Increase1/1 -> OR/1
  Detect Increase/1 -> OR/2, FehlerSpeicher/1(Input)
  OR/1 -> FehlerSpeicher/2(set)
  Compare To Zero/1 -> Detect Increase1/1
  Threshold/1 -> decisionfunction crosses threshold/2
  decision function/1 -> decisionfunction crosses threshold/1, Compare To Zero/1
  decisionfunction crosses threshold/1 -> Detect Increase/1

== system AVE_Library/Fault Detection and Isolation/Robust Deviation Detection/FaultDetection/Threshold evaluation3 ==
  decision function : Inport
  Threshold : Inport  Port=2
  Compare To Zero : simulink/Logic and Bit Operations/Compare To Zero  relop===  OutDataTypeStr=boolean
  Detect Decrease : simulink/Logic and Bit Operations/Detect Decrease  vinit=0.0  OutDataTypeStr=boolean
  Detect Increase : simulink/Logic and Bit Operations/Detect Increase  vinit=0.0  OutDataTypeStr=boolean
  Detect Increase1 : simulink/Logic and Bit Operations/Detect Increase  vinit=0.0  OutDataTypeStr=boolean
  Detect Increase2 : simulink/Logic and Bit Operations/Detect Increase  vinit=0.0  OutDataTypeStr=boolean
  FehlerSpeicher : Subsystem  mask(save current signal value){}
      mask help:
      | If set is not zero, the input is feed throug to the output.
      | If set is zero, the output remains the last intput value when set was not zero.
      | Initial value is zero.
  OR : Logic  Operator=OR  AllPortsSameDT=off  OutDataTypeStr=boolean
  decisionfunction crosses threshold : RelationalOperator  OutDataTypeStr=boolean  InputSameDT=off
  pulse if fault detected : Outport  VectorParamsAs1DForOutWhenUnconnected=off
  pulse if fault cleared : Outport  Port=2  VectorParamsAs1DForOutWhenUnconnected=off
  Fault active = true : Outport  Port=3  VectorParamsAs1DForOutWhenUnconnected=off
  wires:
  decisionfunction crosses threshold/1 -> Detect Increase/1
  decision function/1 -> Compare To Zero/1, decisionfunction crosses threshold/1
  Threshold/1 -> decisionfunction crosses threshold/2
  Compare To Zero/1 -> Detect Increase1/1
  OR/1 -> FehlerSpeicher/2(set)
  Detect Increase/1 -> FehlerSpeicher/1(Input), OR/2
  Detect Increase1/1 -> OR/1
  FehlerSpeicher/1(initial=0  saved value) -> Fault active = true/1, Detect Decrease/1, Detect Increase2/1
  Detect Increase2/1 -> pulse if fault detected/1
  Detect Decrease/1 -> pulse if fault cleared/1

== system AVE_Library/Fault Detection and Isolation/Robust Deviation Detection/FaultDetection/Worst Time ==
  decision function : Inport
  current time : Inport  Port=2
  Memory : Memory  InheritSampleTime=on
  Save current signal value initial is zero : Subsystem  mask(save current signal value){}
      mask help:
      | If set is not zero, the input is feed throug to the output.
      | If set is zero, the output remains the last intput value when set was not zero.
      | Initial value is zero.
  Save current signal value initial is zero2 : Subsystem  mask(save current signal value){}
      mask help:
      | If set is not zero, the input is feed throug to the output.
      | If set is zero, the output remains the last intput value when set was not zero.
      | Initial value is zero.
  decisionfunction crosses threshold : RelationalOperator  OutDataTypeStr=boolean  InputSameDT=off
  worst situation : Outport  VectorParamsAs1DForOutWhenUnconnected=off
  wires:
  Memory/1 -> decisionfunction crosses threshold/2
  decision function/1 -> decisionfunction crosses threshold/1, Save current signal value initial is zero/1(Input)
  Save current signal value initial is zero/1(initial=0  saved value) -> Memory/1
  Save current signal value initial is zero2/1(initial=0  saved value) -> worst situation/1
  current time/1 -> Save current signal value initial is zero2/1(Input)
  decisionfunction crosses threshold/1 -> Save current signal value initial is zero/2(set), Save current signal value initial is zero2/2(set)

== system AVE_Library/Fault Detection and Isolation/Robust Deviation Detection/FaultDetection/cumulative sum calculation1 ==
  LogLikRat : Inport
  Threshold : Inport  Port=2
  Enable : EnablePort
  Constant : Constant  Value=0
  Memory : Memory  InheritSampleTime=on
  Saturation Dynamic : simulink/Discontinuities/Saturation Dynamic  OutMin=[]  OutMax=[]  OutDataTypeStr=Inherit: Same as second input  OutDataType=fixdt(1, 16)  OutScaling=2^-10  DoSatur=off
  Sum : Sum  Inputs=|++
  CUSUM : Outport  VectorParamsAs1DForOutWhenUnconnected=off
  wires:
  Constant/1 -> Saturation Dynamic/3
  Threshold/1 -> Saturation Dynamic/1
  Saturation Dynamic/1 -> CUSUM/1, Memory/1
  Sum/1 -> Saturation Dynamic/2
  LogLikRat/1 -> Sum/2
  Memory/1 -> Sum/1

== system AVE_Library/Fault Detection and Isolation/Robust Deviation Detection/FaultDetection/cumulative sum calculation2 ==
  LogLikRat : Inport
  Threshold : Inport  Port=2
  Enable : EnablePort
  Constant : Constant  Value=0
  Memory : Memory  InheritSampleTime=on
  Saturation Dynamic : simulink/Discontinuities/Saturation Dynamic  OutMin=[]  OutMax=[]  OutDataTypeStr=Inherit: Same as second input  OutDataType=fixdt(1, 16)  OutScaling=2^-10  DoSatur=off
  Sum : Sum  Inputs=|++
  CUSUM : Outport  VectorParamsAs1DForOutWhenUnconnected=off
  wires:
  Memory/1 -> Sum/1
  LogLikRat/1 -> Sum/2
  Sum/1 -> Saturation Dynamic/2
  Saturation Dynamic/1 -> Memory/1, CUSUM/1
  Threshold/1 -> Saturation Dynamic/1
  Constant/1 -> Saturation Dynamic/3

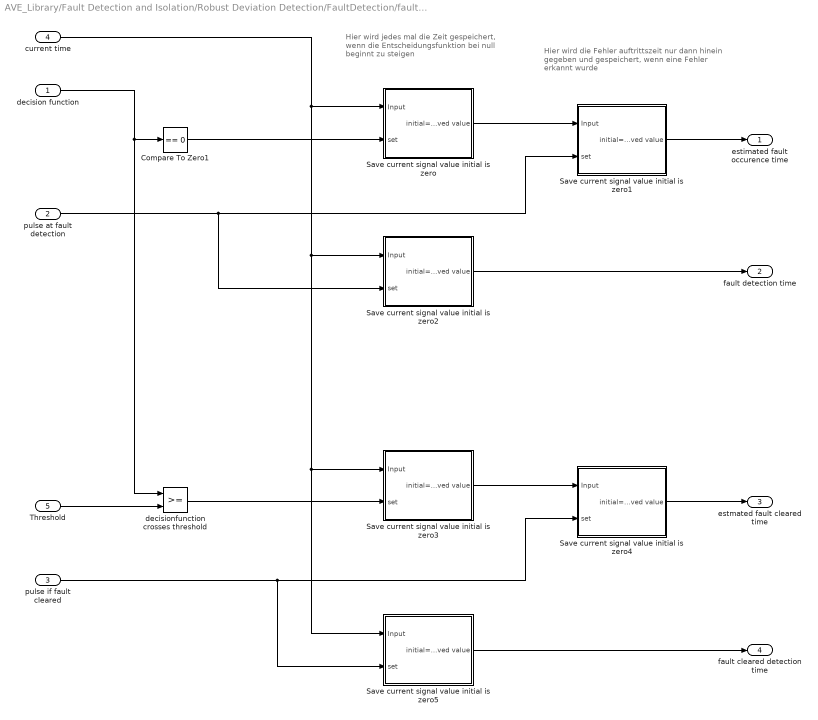
== system AVE_Library/Fault Detection and Isolation/Robust Deviation Detection/FaultDetection/fault occurence time1 ==
  note: Hier wird die Fehler auftrittszeit nur dann hinein
      | gegeben und gespeichert, wenn eine Fehler
      | erkannt wurde
  note: Hier wird jedes mal die Zeit gespeichert,
      | wenn die Entscheidungsfunktion bei null
      | beginnt zu steigen
  decision function : Inport
  pulse at fault detection : Inport  Port=2
  pulse if fault cleared : Inport  Port=3
  current time : Inport  Port=4
  Threshold : Inport  Port=5
  Compare To Zero1 : simulink/Logic and Bit Operations/Compare To Zero  relop===  OutDataTypeStr=boolean
  Save current signal value initial is zero : Subsystem  mask(save current signal value){}
      mask help:
      | If set is not zero, the input is feed throug to the output.
      | If set is zero, the output remains the last intput value when set was not zero.
      | Initial value is zero.
  Save current signal value initial is zero1 : Subsystem  mask(save current signal value){}
      mask help:
      | If set is not zero, the input is feed throug to the output.
      | If set is zero, the output remains the last intput value when set was not zero.
      | Initial value is zero.
  Save current signal value initial is zero2 : Subsystem  mask(save current signal value){}
      mask help:
      | If set is not zero, the input is feed throug to the output.
      | If set is zero, the output remains the last intput value when set was not zero.
      | Initial value is zero.
  Save current signal value initial is zero3 : Subsystem  mask(save current signal value){}
      mask help:
      | If set is not zero, the input is feed throug to the output.
      | If set is zero, the output remains the last intput value when set was not zero.
      | Initial value is zero.
  Save current signal value initial is zero4 : Subsystem  mask(save current signal value){}
      mask help:
      | If set is not zero, the input is feed throug to the output.
      | If set is zero, the output remains the last intput value when set was not zero.
      | Initial value is zero.
  Save current signal value initial is zero5 : Subsystem  mask(save current signal value){}
      mask help:
      | If set is not zero, the input is feed throug to the output.
      | If set is zero, the output remains the last intput value when set was not zero.
      | Initial value is zero.
  decisionfunction crosses threshold : RelationalOperator  OutDataTypeStr=boolean  InputSameDT=off
  estimated fault occurence time : Outport  VectorParamsAs1DForOutWhenUnconnected=off
  fault detection time : Outport  Port=2  VectorParamsAs1DForOutWhenUnconnected=off
  estmated fault cleared time : Outport  Port=3  VectorParamsAs1DForOutWhenUnconnected=off
  fault cleared detection time : Outport  Port=4  VectorParamsAs1DForOutWhenUnconnected=off
  wires:
  Save current signal value initial is zero5/1(initial=0  saved value) -> fault cleared detection time/1
  Threshold/1 -> decisionfunction crosses threshold/2
  decisionfunction crosses threshold/1 -> Save current signal value initial is zero3/2(set)
  current time/1 -> Save current signal value initial is zero/1(Input), Save current signal value initial is zero2/1(Input), Save current signal value initial is zero3/1(Input), Save current signal value initial is zero5/1(Input)
  Save current signal value initial is zero4/1(initial=0  saved value) -> estmated fault cleared time/1
  pulse if fault cleared/1 -> Save current signal value initial is zero4/2(set), Save current signal value initial is zero5/2(set)
  Save current signal value initial is zero3/1(initial=0  saved value) -> Save current signal value initial is zero4/1(Input)
  Save current signal value initial is zero2/1(initial=0  saved value) -> fault detection time/1
  Save current signal value initial is zero/1(initial=0  saved value) -> Save current signal value initial is zero1/1(Input)
  pulse at fault detection/1 -> Save current signal value initial is zero1/2(set), Save current signal value initial is zero2/2(set)
  Save current signal value initial is zero1/1(initial=0  saved value) -> estimated fault occurence time/1
  decision function/1 -> Compare To Zero1/1, decisionfunction crosses threshold/1
  Compare To Zero1/1 -> Save current signal value initial is zero/2(set)
